simulink model "B5_simulation_paparazzi"  (R2021b)
settings: Solver=VariableStepAuto  StartTime=0.0  StopTime=5.5  FixedStep=0.002  RelTol=1e-3
values from neighbouring files (symbols this model uses):
  coef_sim_1 = tf_des_d.Denominator{1}(2)    [A11_setup_script_pprz.m]    (also in A1_setup_script.m; A6_slow_actuator.m)
  coef_sim_2 = tf_des_d.Numerator{1}(2)    [A11_setup_script_pprz.m]    (also in A1_setup_script.m; A6_slow_actuator.m)
  coeff = 1    [A11_setup_script_pprz.m]    (also in A12_sim_multi_run.m = coeff_list(i))
  doublet_mag = - 0.15    (= -0.15)    [A11_setup_script_pprz.m]    (also in A1_setup_script.m)
  doublet_time = 6    [A11_setup_script_pprz.m]    (also in A1_setup_script.m)
  f_8 = 1    [A11_setup_script_pprz.m]    (also in A1_setup_script.m)
  FILT_CUTOFF = 2*pi*5    (= 31.4159265359)    [A11_setup_script_pprz.m]    (also in A1_setup_script.m)
  FILTER = 1    [A11_setup_script_pprz.m]    (also in A1_setup_script.m)
  G1 = inv(I)*G1_r    [A10_simple_plant.m]    (also in A11_setup_script_pprz.m = G1/scale; A1_setup_script.m = [G1;G1_T])
  G2 = G2/scale    [A11_setup_script_pprz.m]    (also in A1_setup_script.m = (1/sampling_time)*inv(I)*(G2_r))
  h_plate = 0.3    [A11_setup_script_pprz.m]    (also in A1_setup_script.m = 0.16)
  I = eye(3,3)    [A10_simple_plant.m]    (also in A11_setup_script_pprz.m; A1_setup_script.m; A2_B_matrix_generation_symbolic.m = [Ixx 0 0; A3_B_matrix_generation_symbolic_cascaded.m = [Ixx 0 0)
  Iyy = 0.0008    [A11_setup_script_pprz.m]    (also in A1_setup_script.m = 0.0015)
  K = 7    [A11_setup_script_pprz.m]    (also in A1_setup_script.m = 10)
  K_act = 50    [A10_simple_plant.m]    (also in A11_setup_script_pprz.m = 20; A1_setup_script.m = 20)
  K_d = 15    [A11_setup_script_pprz.m]    (also in A1_setup_script.m = 25)
  K_dd = K_act    (= 20)    [A11_setup_script_pprz.m]    (also in A1_setup_script.m)
  K_ec = 50    [A11_setup_script_pprz.m]    (also in A1_setup_script.m = 251)
  K_ec_d = 13    [A11_setup_script_pprz.m]    (also in A1_setup_script.m = 25)
  K_ec_d_u = 1.5    [A11_setup_script_pprz.m]    (also in A1_setup_script.m = 5)
  K_ec_d_v = 1.5    [A11_setup_script_pprz.m]    (also in A1_setup_script.m = 5)
  K_ec_dd = 9    [A11_setup_script_pprz.m]    (also in A1_setup_script.m = 45)
  K_ec_i = 0    [A11_setup_script_pprz.m]    (also in A1_setup_script.m = 380)
  K_ec_u = 1.5    [A11_setup_script_pprz.m]    (also in A1_setup_script.m = 5)
  K_ec_v = 1.5    [A11_setup_script_pprz.m]    (also in A1_setup_script.m = 5)
  K_t = 0.0005    [A10_simple_plant.m]    (also in A11_setup_script_pprz.m = 6.557e-08; A1_setup_script.m = 6.557e-08)
  K_u = 1.0    (= 1)    [A11_setup_script_pprz.m]    (also in A1_setup_script.m = 1.5)
  K_u_d = 2.5    [A11_setup_script_pprz.m]    (also in A1_setup_script.m = 7)
  K_v = 1.0    (= 1)    [A11_setup_script_pprz.m]    (also in A1_setup_script.m = 1.5)
  K_v_d = 2.5    [A11_setup_script_pprz.m]    (also in A1_setup_script.m = 7)
  K_w = 1.0    (= 1)    [A11_setup_script_pprz.m]    (also in A1_setup_script.m = 4.5)
  K_w_d = 2.5    [A11_setup_script_pprz.m]    (also in A1_setup_script.m = 7)
  l_plate = 0.1    [A11_setup_script_pprz.m]    (also in A1_setup_script.m = 0.11)
  m = 0.4    [A10_simple_plant.m]    (also in A11_setup_script_pprz.m; A1_setup_script.m)
  NOISE = 0    [A11_setup_script_pprz.m]    (also in A1_setup_script.m)
  NOISE_ACC = 0.00005    (= 5e-05)    [A11_setup_script_pprz.m]    (also in A1_setup_script.m)
  NOISE_GYRO = 0.00005    (= 5e-05)    [A11_setup_script_pprz.m]    (also in A1_setup_script.m)
  NOISE_RPM = 200    [A11_setup_script_pprz.m]    (also in A1_setup_script.m)
  omega_des = 20.00    (= 20)    [A11_setup_script_pprz.m]    (also in A1_setup_script.m; A6_slow_actuator.m = 49)
  sampling_time = 1/frequency    (= 0.002)    [A11_setup_script_pprz.m]    (also in A12_sim_multi_run.m; A1_setup_script.m; A6_slow_actuator.m)
  scale_8 = 1.6    [A11_setup_script_pprz.m]    (also in A1_setup_script.m)
  start_8 = 2    [A11_setup_script_pprz.m]    (also in A1_setup_script.m)
  start_time = 2    [A11_setup_script_pprz.m]    (also in A1_setup_script.m = 1)
  t_8 = 10    [A11_setup_script_pprz.m]    (also in A1_setup_script.m)
  w_plate = 0.3    [A11_setup_script_pprz.m]    (also in A1_setup_script.m = 0.36)
undefined symbols (not defined in the file or in its folder): DiscIntNeverNeededParam
libraries: simulink x11, cstblocks x9, dspinverses x8, dspmathops x4, dspstat3 x4, aerolibutil x3, sharedutil x2, aerolibanim x1
(part 1 of 5)
settings Model: Creator=pcampolucci  LastModifiedBy=pcampolucci

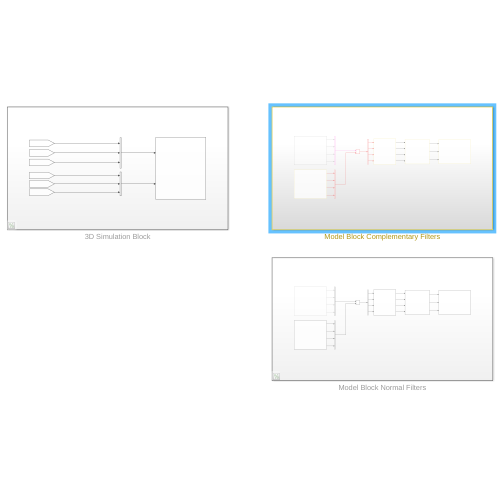
[thumbnail: Simulink's stored preview of the top-level diagram]
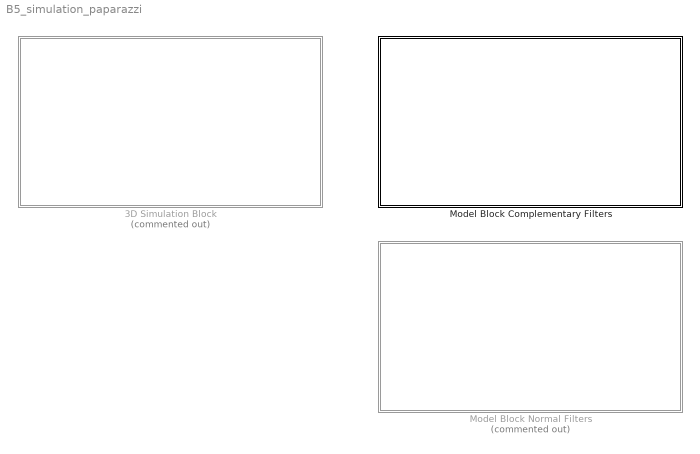
== system B5_simulation_paparazzi ==
  3D Simulation Block : Subsystem  Commented=on
  Model Block Complementary Filters : Subsystem
  Model Block Normal Filters : Subsystem  Commented=on

== system B5_simulation_paparazzi/3D Simulation Block ==
  6DoF Animation : aerolibanim/6DoF Animation  u1=[-4 4 -4 4 -1 1]  u2=0.1  u3=0.3  u4=[0 0 0]  u5=Fly alongside  u6=[5 5 -4]  u7=10  u8=on
  Vector Concatenate : Concatenate  NumInputs=3
  Vector Concatenate1 : Concatenate  NumInputs=3
  wires:
  [psi] -> Vector Concatenate/3
  Vector Concatenate1/1 -> 6DoF Animation/1
  Vector Concatenate/1 -> 6DoF Animation/2
  [X_cont] -> Vector Concatenate1/1
  [Y_cont] -> Vector Concatenate1/2
  [theta] -> Vector Concatenate/2
  [phi] -> Vector Concatenate/1
  [Z_cont] -> Vector Concatenate1/3

== system B5_simulation_paparazzi/Model Block Complementary Filters ==
  Continuous Actuator Dynamics : Subsystem
  Demux : Demux
  Extended INDI : Subsystem
  Force and Moment Calculation : Subsystem
      mask Display: image('/home/pcampolucci/asc-indi-simulator/media/bebop.jpg'); % Use "Edit Image" on toolstrip to change.
  Manual Switch : ManualSwitch
  Mux1 : Mux
  Mux4 : Mux
  Plant and State Estimation : Subsystem
  Simple INDI : Subsystem  Commented=on
  wires:
  Demux/2 -> Continuous Actuator Dynamics/2(Motor_2_omega_input)
  Demux/4 -> Continuous Actuator Dynamics/4(Motor_4_omega_input)
  Continuous Actuator Dynamics/1(omega_1) -> Force and Moment Calculation/1(omega_1)
  Continuous Actuator Dynamics/4(omega_4) -> Force and Moment Calculation/4(omega_4)
  Demux/1 -> Continuous Actuator Dynamics/1(Motor_1_omega_input)
  Force and Moment Calculation/1(Moments in body frame) -> Plant and State Estimation/1(Moments in body frame)
  Continuous Actuator Dynamics/3(omega_3) -> Force and Moment Calculation/3(omega_3)
  Continuous Actuator Dynamics/2(omega_2) -> Force and Moment Calculation/2(omega_2)
  Demux/3 -> Continuous Actuator Dynamics/3(Motor_3_omega_input)
  Force and Moment Calculation/2(Forces in earth frame) -> Plant and State Estimation/2(Forces in earth frame)
  Extended INDI/2(Motor_2_omega_input) -> Mux4/2
  Extended INDI/1(Motor_1_omega_input) -> Mux4/1
  Extended INDI/3(Motor_3_omega_input) -> Mux4/3
  Extended INDI/4(Motor_4_omega_input) -> Mux4/4
  Force and Moment Calculation/3(Collective Thrust) -> Plant and State Estimation/3(Collective Thrust)
  Mux4/1 -> Manual Switch/1
  Manual Switch/1 -> Demux/1
  Simple INDI/1(Motor_1_omega_input) -> Mux1/1
  Simple INDI/2(Motor_2_omega_input) -> Mux1/2
  Simple INDI/3(Motor_3_omega_input) -> Mux1/3
  Simple INDI/4(Motor_4_omega_input) -> Mux1/4
  Mux1/1 -> Manual Switch/2

== system B5_simulation_paparazzi/Model Block Normal Filters ==
  Continuous Actuator Dynamics : Subsystem
  Demux : Demux
  Extended INDI : Subsystem  Commented=on
  Force and Moment Calculation : Subsystem
      mask Display: image('/home/pcampolucci/asc-indi-simulator/media/bebop.jpg'); % Use "Edit Image" on toolstrip to change.
  Manual Switch : ManualSwitch  CurrentSetting=0
  Mux1 : Mux
  Mux4 : Mux
  Plant and State Estimation : Subsystem
  Simple INDI : Subsystem
  wires:
  Demux/2 -> Continuous Actuator Dynamics/2(Motor_2_omega_input)
  Demux/4 -> Continuous Actuator Dynamics/4(Motor_4_omega_input)
  Continuous Actuator Dynamics/1(omega_1) -> Force and Moment Calculation/1(omega_1)
  Continuous Actuator Dynamics/4(omega_4) -> Force and Moment Calculation/4(omega_4)
  Demux/1 -> Continuous Actuator Dynamics/1(Motor_1_omega_input)
  Force and Moment Calculation/1(Moments in body frame) -> Plant and State Estimation/1(Moments in body frame)
  Continuous Actuator Dynamics/3(omega_3) -> Force and Moment Calculation/3(omega_3)
  Continuous Actuator Dynamics/2(omega_2) -> Force and Moment Calculation/2(omega_2)
  Demux/3 -> Continuous Actuator Dynamics/3(Motor_3_omega_input)
  Force and Moment Calculation/2(Forces in earth frame) -> Plant and State Estimation/2(Forces in earth frame)
  Extended INDI/2(Motor_2_omega_input) -> Mux4/2
  Extended INDI/1(Motor_1_omega_input) -> Mux4/1
  Extended INDI/3(Motor_3_omega_input) -> Mux4/3
  Extended INDI/4(Motor_4_omega_input) -> Mux4/4
  Force and Moment Calculation/3(Collective Thrust) -> Plant and State Estimation/3(Collective Thrust)
  Mux4/1 -> Manual Switch/1
  Manual Switch/1 -> Demux/1
  Simple INDI/1(Motor_1_omega_input) -> Mux1/1
  Simple INDI/2(Motor_2_omega_input) -> Mux1/2
  Simple INDI/3(Motor_3_omega_input) -> Mux1/3
  Simple INDI/4(Motor_4_omega_input) -> Mux1/4
  Mux1/1 -> Manual Switch/2

== system B5_simulation_paparazzi/Model Block Complementary Filters/Continuous Actuator Dynamics ==
  Motor_1_omega_input : Inport
  Motor_2_omega_input : Inport  Port=2
  Motor_3_omega_input : Inport  Port=3
  Motor_4_omega_input : Inport  Port=4
  Demux : Demux
  Discrete Transfer Fcn{1..4} (4 alike) : DiscreteTransferFcn  Numerator=[coef_sim_2]  Denominator=[1 coef_sim_1]  SampleTime=sampling_time
  Mux : Mux
  Noise RPM : Subsystem
  Sum : Sum  Inputs=|++
  Transfer Fcn{,1..3} (4 alike) : TransferFcn  Numerator=[omega_des]  Denominator=[1 omega_des]
  omega_1 : Outport
  omega_2 : Outport  Port=2
  omega_3 : Outport  Port=3
  omega_4 : Outport  Port=4
  tag scope: omega_1_f=global, omega_2_f=global, omega_3_f=global, omega_4_f=global
  wires:
  Transfer Fcn3/1 -> omega_4/1  "omega_4"
  Motor_4_omega_input/1 -> Transfer Fcn3/1, Discrete Transfer Fcn4/1  "omega_4_in"
  Motor_3_omega_input/1 -> Transfer Fcn2/1, Discrete Transfer Fcn3/1  "omega_3_in"
  Transfer Fcn1/1 -> omega_2/1  "omega_2"
  Discrete Transfer Fcn2/1 -> Mux/1
  Motor_2_omega_input/1 -> Transfer Fcn1/1, Discrete Transfer Fcn1/1  "omega_2_in"
  Demux/2 -> [omega_2_f]  "omega_2_est"
  Motor_1_omega_input/1 -> Discrete Transfer Fcn2/1, Transfer Fcn/1  "omega_1_in"
  Transfer Fcn/1 -> omega_1/1  "omega_1"
  Demux/4 -> [omega_4_f]  "omega_4_est"
  Discrete Transfer Fcn4/1 -> Mux/4
  Discrete Transfer Fcn1/1 -> Mux/2
  Discrete Transfer Fcn3/1 -> Mux/3
  Transfer Fcn2/1 -> omega_3/1  "omega_3"
  Demux/1 -> [omega_1_f]  "omega_1_est"
  Demux/3 -> [omega_3_f]  "omega_3_est"
  Mux/1 -> Sum/1  "pqr_measured"
  Noise RPM/1(Out) -> Sum/2
  Sum/1 -> Demux/1

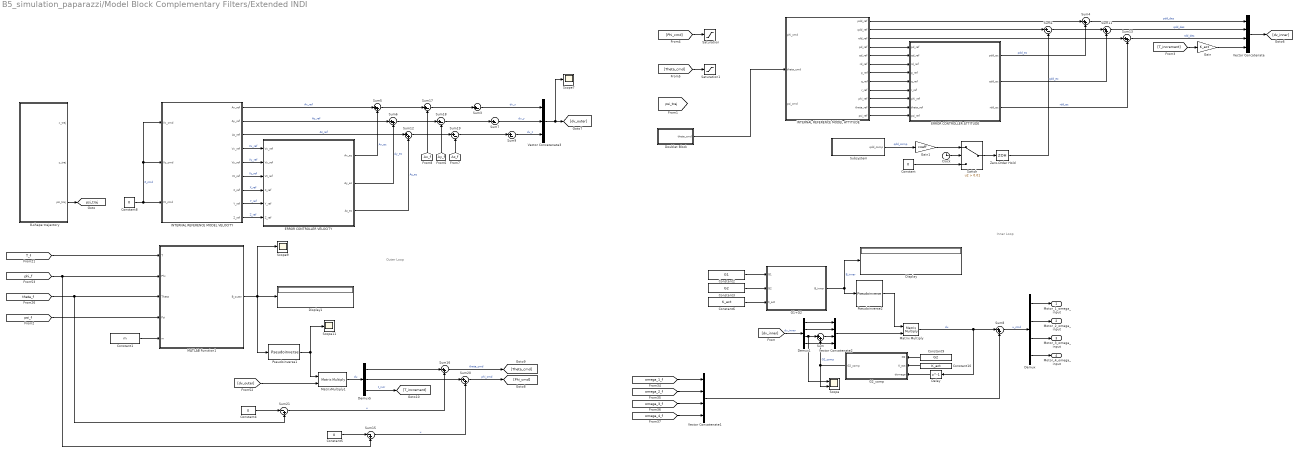
== system B5_simulation_paparazzi/Model Block Complementary Filters/Extended INDI ==
  note: Inner Loop
  note: Outer Loop
  8-shape trajectory : Subsystem
  Clock : Clock
  Constant : Constant  Value=0  SampleTime=sampling_time
  Constant1 : Constant  Value=m  SampleTime=sampling_time
  Constant10 : Constant  Value=K_act  SampleTime=sampling_time
  Constant2 : Constant  Value=G1  SampleTime=sampling_time
  Constant3 : Constant  Value=G2  SampleTime=sampling_time
  Constant4 : Constant  Value=0
  Constant5 : Constant  Value=0
  Constant6 : Constant  Value=K_act  SampleTime=sampling_time
  Constant8 : Constant  Value=0  SampleTime=sampling_time
  Constant9 : Constant  Value=G2  SampleTime=sampling_time
  Delay : Delay  DelayLength=1
  Demux : Demux
  Demux1 : Demux
  Demux5 : Demux  Outputs=3
  Display : Display
  Display1 : Display
  Doublet Block : Subsystem
  ERROR CONTROLLER ATTITUDE : Subsystem
  ERROR CONTROLLER VELOCITY : Subsystem
  G1+G2 : MATLAB Function  TreatAsAtomicUnit=on
  G2_comp : MATLAB Function  TreatAsAtomicUnit=on
  Gain : Gain  Gain=K_act
  Gain1 : Gain  Gain=coeff
  INTERNAL REFERENCE MODEL ATTITUDE : Subsystem
  INTERNAL REFERENCE MODEL VELOCITY : Subsystem
  MATLAB Function1 : MATLAB Function  TreatAsAtomicUnit=on
  Matrix Multiply : Product  Multiplication=Matrix(*)
  MatrixMultiply1 : Product  Multiplication=Matrix(*)
  Pseudoinverse1 : dspinverses/Pseudoinverse  wanterr=off  SimulateUsing=Interpreted execution
      settings: SourceProductBaseCode=DS
  Pseudoinverse2 : dspinverses/Pseudoinverse  wanterr=off  SimulateUsing=Interpreted execution
      settings: SourceProductBaseCode=DS
  Saturation : Saturate
  Saturation1 : Saturate
  Scope : Scope  NumInputPorts=2
  Scope11 : Scope
  Scope7 : Scope
  Scope9 : Scope
  Subsystem : Subsystem
  Sum{,4..6,8,11..13,16,20} (10 alike) : Sum  Inputs=|++
  Sum{1,3,7,9,17..19} (7 alike) : Sum  Inputs=|+-
  Sum15 : Sum  Inputs=|-+
  Sum21 : Sum  Inputs=|-+
  Switch : Switch  Criteria=u2 > Threshold  Threshold=0.01
  Vector Concatenate : Concatenate  NumInputs=4
  Vector Concatenate1 : Concatenate  NumInputs=4
  Vector Concatenate2 : Concatenate  NumInputs=4
  Vector Concatenate3 : Concatenate  NumInputs=3
  Zero-Order Hold : ZeroOrderHold  SampleTime=sampling_time
  Motor_1_omega_input : Outport
  Motor_2_omega_input : Outport  Port=2
  Motor_3_omega_input : Outport  Port=3
  Motor_4_omega_input : Outport  Port=4
  tag scope: psi_traj=global
  wires:
  G1+G2/1(B_inner) -> Pseudoinverse2/1, Display/1  "B_inner"
  Vector Concatenate/1 -> [dv_inner]
  Matrix Multiply/1 -> Delay/1, Sum8/1  "du"
  Demux/1 -> Motor_1_omega_input/1
  [omega_4_f] -> Vector Concatenate1/4
  [omega_2_f] -> Vector Concatenate1/2
  Demux/3 -> Motor_3_omega_input/1
  Sum8/1 -> Demux/1  "u_cmd"
  Pseudoinverse2/1 -> Matrix Multiply/1
  [omega_1_f] -> Vector Concatenate1/1
  Demux/2 -> Motor_2_omega_input/1
  Demux/4 -> Motor_4_omega_input/1
  [omega_3_f] -> Vector Concatenate1/3
  INTERNAL REFERENCE MODEL VELOCITY/5(Vy_ref) -> ERROR CONTROLLER VELOCITY/2(Vy_ref)  "Vy_ref"
  Constant4/1 -> Sum21/1
  Sum16/1 -> [Theta_cmd]  "theta_cmd"
  Sum9/1 -> Vector Concatenate3/3  "dv_z"
  INTERNAL REFERENCE MODEL VELOCITY/2(Ay_ref) -> Sum6/1  "Ay_ref"
  Sum21/1 -> Sum16/2  "u"
  INTERNAL REFERENCE MODEL VELOCITY/6(Vz_ref) -> ERROR CONTROLLER VELOCITY/3(Vz_ref)  "Vz_ref"
  INTERNAL REFERENCE MODEL VELOCITY/4(Vx_ref) -> ERROR CONTROLLER VELOCITY/1(Vx_ref)  "Vx_ref"
  ERROR CONTROLLER VELOCITY/2(Ay_ec) -> Sum6/2  "Ay_ec"
  Sum7/1 -> Vector Concatenate3/2  "dv_y"
  ERROR CONTROLLER VELOCITY/1(Ax_ec) -> Sum5/2  "Ax_ec"
  Sum3/1 -> Vector Concatenate3/1  "dv_x"
  ERROR CONTROLLER VELOCITY/3(Az_ec) -> Sum12/2  "Az_ec"
  Sum12/1 -> Sum19/1
  Constant8/1 -> INTERNAL REFERENCE MODEL VELOCITY/2(Vy_cmd), INTERNAL REFERENCE MODEL VELOCITY/1(Vx_cmd), INTERNAL REFERENCE MODEL VELOCITY/3(Vz_cmd)  "Z_cmd"
  Pseudoinverse1/1 -> Scope11/1, MatrixMultiply1/1
  Sum15/1 -> Sum20/2  "u"
  Vector Concatenate3/1 -> Scope7/1, [dv_outer]
  INTERNAL REFERENCE MODEL VELOCITY/1(Ax_ref) -> Sum5/1  "Ax_ref"
  INTERNAL REFERENCE MODEL VELOCITY/3(Az_ref) -> Sum12/1  "Az_ref"
  Sum20/1 -> [Phi_cmd]  "phi_cmd"
  [T_f] -> MATLAB Function1/1(T)
  Sum6/1 -> Sum18/1
  Constant5/1 -> Sum15/1
  [dv_outer] -> MatrixMultiply1/2
  MATLAB Function1/1(B_outer) -> Scope9/1, Display1/1, Pseudoinverse1/1
  Demux5/3 -> [T_increment]  "t_incr"
  MatrixMultiply1/1 -> Demux5/1  "du"
  [T_increment] -> Gain/1
  [Ax_f] -> Sum17/2
  [Ay_f] -> Sum18/2
  [Az_f] -> Sum19/2
  [Phi_cmd] -> Saturation/1
  [theta_f] -> Sum21/2, MATLAB Function1/3(Theta)
  [phi_f] -> Sum15/2, MATLAB Function1/2(Phi)
  INTERNAL REFERENCE MODEL ATTITUDE/4(pd_ref) -> ERROR CONTROLLER ATTITUDE/1(pd_ref)
  INTERNAL REFERENCE MODEL ATTITUDE/7(p_ref) -> ERROR CONTROLLER ATTITUDE/4(p_ref)
  ERROR CONTROLLER ATTITUDE/3(rdd_ec) -> Sum13/2  "rdd_ec"
  ERROR CONTROLLER ATTITUDE/2(qdd_ec) -> Sum11/2  "qdd_ec"
  INTERNAL REFERENCE MODEL ATTITUDE/5(qd_ref) -> ERROR CONTROLLER ATTITUDE/2(qd_ref)
  INTERNAL REFERENCE MODEL ATTITUDE/11(theta_ref) -> ERROR CONTROLLER ATTITUDE/8(theta_ref)
  INTERNAL REFERENCE MODEL ATTITUDE/1(pdd_ref) -> Sum4/1
  INTERNAL REFERENCE MODEL ATTITUDE/8(q_ref) -> ERROR CONTROLLER ATTITUDE/5(q_ref)
  ERROR CONTROLLER ATTITUDE/1(pdd_ec) -> Sum4/2  "pdd_ec"
  INTERNAL REFERENCE MODEL ATTITUDE/6(rd_ref) -> ERROR CONTROLLER ATTITUDE/3(rd_ref)
  INTERNAL REFERENCE MODEL ATTITUDE/10(phi_ref) -> ERROR CONTROLLER ATTITUDE/7(phi_ref)
  INTERNAL REFERENCE MODEL ATTITUDE/12(psi_ref) -> ERROR CONTROLLER ATTITUDE/9(psi_ref)
  INTERNAL REFERENCE MODEL ATTITUDE/9(r_ref) -> ERROR CONTROLLER ATTITUDE/6(r_ref)
  Sum13/1 -> Vector Concatenate/3  "rdd_des"
  Sum4/1 -> Vector Concatenate/1  "pdd_des"
  Sum11/1 -> Vector Concatenate/2  "qdd_des"
  Gain/1 -> Vector Concatenate/4
  Constant3/1 -> G1+G2/2(G2)
  Constant6/1 -> G1+G2/3(K_act)
  Constant2/1 -> G1+G2/1(G1)
  Constant9/1 -> G2_comp/1(G2)
  Constant10/1 -> G2_comp/2(K_act)
  [dv_inner] -> Demux1/1  "dv_inner"
  Sum/1 -> Vector Concatenate2/3
  Demux1/3 -> Scope/1, Sum/1
  Demux1/2 -> Vector Concatenate2/2
  Demux1/1 -> Vector Concatenate2/1
  Demux1/4 -> Vector Concatenate2/4
  Vector Concatenate2/1 -> Matrix Multiply/2
  G2_comp/1(G2_comp) -> Sum/2, Scope/2  "G2_comp"
  Sum5/1 -> Sum17/1
  INTERNAL REFERENCE MODEL ATTITUDE/2(qdd_ref) -> Sum1/1
  8-shape trajectory/3(psi_traj) -> [psi_traj]
  [Theta_cmd] -> Saturation1/1
  Sum17/1 -> Sum3/1
  Sum18/1 -> Sum7/1
  Sum19/1 -> Sum9/1
  Constant1/1 -> MATLAB Function1/5(m)
  Demux5/2 -> Sum20/1
  Demux5/1 -> Sum16/1
  [psi_f] -> MATLAB Function1/4(Psi)
  Clock/1 -> Switch/2
  Constant/1 -> Switch/3
  Switch/1 -> Zero-Order Hold/1
  INTERNAL REFERENCE MODEL VELOCITY/7(X_ref) -> ERROR CONTROLLER VELOCITY/4(X_ref)  "X_ref"
  INTERNAL REFERENCE MODEL VELOCITY/8(Y_ref) -> ERROR CONTROLLER VELOCITY/5(Y_ref)  "Y_ref"
  INTERNAL REFERENCE MODEL VELOCITY/9(Z_ref) -> ERROR CONTROLLER VELOCITY/6(Z_ref)  "Z_ref"
  Doublet Block/1(theta_cmd) -> INTERNAL REFERENCE MODEL ATTITUDE/2(theta_cmd)
  INTERNAL REFERENCE MODEL ATTITUDE/3(rdd_ref) -> Sum13/1
  Subsystem/1(qdd_comp) -> Gain1/1  "qdd_comp"
  Sum1/1 -> Sum11/1
  Zero-Order Hold/1 -> Sum1/2
  Gain1/1 -> Switch/1
  Vector Concatenate1/1 -> Sum8/2
  Delay/1 -> G2_comp/3(domega)

== system B5_simulation_paparazzi/Model Block Complementary Filters/Force and Moment Calculation ==
  omega_1 : Inport
  omega_2 : Inport  Port=2
  omega_3 : Inport  Port=3
  omega_4 : Inport  Port=4
  Add : Sum
  Add1 : Sum
  Constant : Constant  Value=0
  Constant1 : Constant  Value=sampling_time  SampleTime=sampling_time
  Constant2 : Constant  Value=G1  SampleTime=sampling_time
  Constant3 : Constant  Value=G2  SampleTime=sampling_time
  Constant5 : Constant  Value=I  SampleTime=sampling_time
  Derivative : Derivative
  Drag Plate Aerodynamics : Subsystem
  Forces due to thrust : MATLAB Function  TreatAsAtomicUnit=on
  Gain : Gain  Gain=0.09
  Gain1 : Gain  Gain=0.09
  Moments due to thrust : MATLAB Function  TreatAsAtomicUnit=on
  Mux : Mux
  Mux1 : Mux  Inputs=3
  Sum : Sum  Inputs=|++
  Moments in body frame : Outport
  Forces in earth frame : Outport  Port=2
  Collective Thrust : Outport  Port=3
  wires:
  Moments due to thrust/1(M_t) -> Add1/2  "thrust_moment_in"
  Constant2/1 -> Forces due to thrust/3(G1), Moments due to thrust/3(G1)
  Constant3/1 -> Moments due to thrust/4(G2)
  omega_4/1 -> Mux/4
  omega_3/1 -> Mux/3
  omega_2/1 -> Mux/2
  omega_1/1 -> Mux/1
  Mux/1 -> Derivative/1, Forces due to thrust/1(omega), Moments due to thrust/1(omega)
  Derivative/1 -> Moments due to thrust/2(omega_dot)
  Constant1/1 -> Moments due to thrust/5(sampling_time)
  [R_bg] -> Forces due to thrust/2(R_bg)
  Forces due to thrust/1(F_t_e) -> Add/2  "thrust_earth"
  Forces due to thrust/2(F_t_b) -> Collective Thrust/1  "thrust_body"
  Add/1 -> Forces in earth frame/1
  Add1/1 -> Moments in body frame/1  "full_moment_in"
  Constant5/1 -> Moments due to thrust/6(I)
  Drag Plate Aerodynamics/1(aero_moment) -> Add1/1  "aero_moment_in"
  Constant/1 -> Mux1/3, Mux1/1
  [theta_cont] -> Gain/1
  [phi_cont] -> Gain1/1
  Gain/1 -> Sum/1
  Gain1/1 -> Sum/2
  Sum/1 -> Mux1/2
  Mux1/1 -> ?  "dummy_moment"

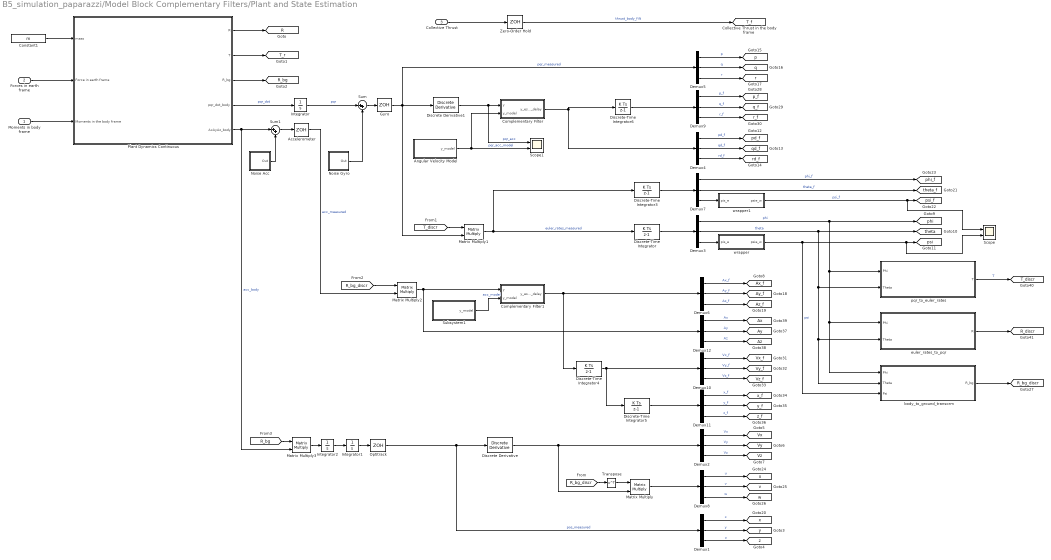
== system B5_simulation_paparazzi/Model Block Complementary Filters/Plant and State Estimation ==
  Moments in body frame : Inport
  Forces in earth frame : Inport  Port=2
  Collective Thrust : Inport  Port=3
  Accelerometer : ZeroOrderHold  SampleTime=sampling_time
  Angular Velocity Model : Subsystem
  Complementary Filter : Subsystem
  Complementary Filter1 : Subsystem
  Constant1 : Constant  Value=m  SampleTime=sampling_time
  Demux{1..12} (12 alike) : Demux  Outputs=3
  Discrete Derivative : simulink/Discrete/Discrete Derivative  gainval=1.0  ICPrevScaledInput=0.0  OutMin=[]  OutMax=[]  OutDataType=fixdt(1, 16)  OutScaling=2^-10  DoSatur=off
  Discrete Derivative1 : simulink/Discrete/Discrete Derivative  gainval=1.0  ICPrevScaledInput=0.0  OutMin=[]  OutMax=[]  OutDataType=fixdt(1, 16)  OutScaling=2^-10  DoSatur=off
  Discrete-Time Integrator{,3..5} (4 alike) : DiscreteIntegrator  SampleTime=sampling_time  ICPrevOutput=DiscIntNeverNeededParam  ICPrevScaledInput=DiscIntNeverNeededParam
  Discrete-Time Integrator6 : DiscreteIntegrator  SampleTime=-1  ICPrevOutput=DiscIntNeverNeededParam  ICPrevScaledInput=DiscIntNeverNeededParam
  Gyro : ZeroOrderHold  SampleTime=sampling_time
  Integrator : Integrator
  Integrator1 : Integrator
  Integrator2 : Integrator
  Matrix Multiply{,1..3} (4 alike) : Product  Multiplication=Matrix(*)
  Noise Acc : Subsystem
  Noise Gyro : Subsystem
  Optitrack : ZeroOrderHold  SampleTime=sampling_time
  Plant Dynamics Continuous : Subsystem
  Scope : Scope  NumInputPorts=2
  Scope1 : Scope  NumInputPorts=2
  Subsystem1 : Subsystem
  Sum : Sum  Inputs=|++
  Sum1 : Sum  Inputs=|++
  Transpose : Math  Operator=transpose  SaturateOnIntegerOverflow=on
  Zero-Order Hold : ZeroOrderHold  SampleTime=sampling_time
  body_to_ground_transorm : MATLAB Function  Description=|  TreatAsAtomicUnit=on
      | This function computes the rotational matrix to pass from the body frame to the world frame. 
      | Takes as inpout the euler angles.
  euler_rates_to_pqr : MATLAB Function  TreatAsAtomicUnit=on
  pqr_to_euler_rates : MATLAB Function  TreatAsAtomicUnit=on
  wrapper : MATLAB Function  TreatAsAtomicUnit=on
  wrapper1 : MATLAB Function  TreatAsAtomicUnit=on
  tag scope: Ax=global, Ax_f=global, Ay=global, Ay_f=global, Az=global, Az_f=global, R=global, R_bg=global, R_bg_discr=global, R_discr=global, T_discr=global, T_f=global, T_r=global, Vx=global, Vx_f=global, Vy=global, Vy_f=global, Vz=global, Vz_f=global, p=global, p_f=global, pd_f=global, phi=global, phi_f=global, psi=global, psi_f=global, q=global, q_f=global, qd_f=global, r=global, r_f=global, rd_f=global, theta=global, theta_f=global, u=global, v=global, w=global, x=global, x_f=global, y=global, y_f=global, z=global, z_f=global
  wires:
  Demux3/2 -> euler_rates_to_pqr/2(Theta), body_to_ground_transorm/2(Theta), pqr_to_euler_rates/2(Theta), [theta]  "theta"
  Demux4/1 -> [pd_f]  "pd_f"
  Demux3/1 -> body_to_ground_transorm/1(Phi), euler_rates_to_pqr/1(Phi), pqr_to_euler_rates/1(Phi), [phi]  "phi"
  Demux4/2 -> [qd_f]  "qd_f"
  Demux3/3 -> wrapper/1(pis_e)
  Discrete-Time Integrator/1 -> Demux3/1
  Demux5/2 -> [q]  "q"
  Demux5/1 -> [p]  "p"
  Plant Dynamics Continuous/4(pqr_dot_body) -> Integrator/1  "pqr_dot"
  Demux5/3 -> [r]  "r"
  Integrator/1 -> Sum/1  "pqr"
  Complementary Filter/1(y_est_no_delay) -> Discrete-Time Integrator6/1, Demux4/1
  Demux4/3 -> [rd_f]  "rd_f"
  Moments in body frame/1 -> Plant Dynamics Continuous/3(Moments in the body frame)
  Constant1/1 -> Plant Dynamics Continuous/1(mass)
  Forces in earth frame/1 -> Plant Dynamics Continuous/2(Force in earth frame)
  Plant Dynamics Continuous/1(R) -> [R]
  Plant Dynamics Continuous/2(T) -> [T_r]
  Plant Dynamics Continuous/3(R_bg) -> [R_bg]
  Demux2/2 -> [Vy]  "Vy"
  Demux6/2 -> [Ay_f]  "Ay_f"
  Discrete Derivative/1 -> Demux2/1, Matrix Multiply/2
  Demux6/1 -> [Ax_f]  "Ax_f"
  Accelerometer/1 -> Matrix Multiply2/2  "acc_measured"
  Demux2/1 -> [Vx]  "Vx"
  Demux1/2 -> [y]  "y"
  Demux1/1 -> [x]  "x"
  Demux1/3 -> [z]  "z"
  Demux6/3 -> [Az_f]  "Az_f"
  Demux2/3 -> [Vz]  "Vz"
  Plant Dynamics Continuous/5(AxAyAz_body) -> Matrix Multiply3/2, Sum1/1  "acc_body"
  Demux7/3 -> wrapper1/1(pis_e)
  Demux7/1 -> [phi_f]  "phi_f"
  Demux7/2 -> [theta_f]  "theta_f"
  Discrete-Time Integrator3/1 -> Demux7/1
  [R_bg_discr] -> Transpose/1
  Transpose/1 -> Matrix Multiply/1
  Demux8/2 -> [v]  "v"
  Demux8/1 -> [u]  "u"
  Demux8/3 -> [w]  "w"
  Matrix Multiply/1 -> Demux8/1
  Zero-Order Hold/1 -> [T_f]  "thrust_body_filt"
  Collective Thrust/1 -> Zero-Order Hold/1
  Demux9/3 -> [r_f]  "r_f"
  Demux9/1 -> [p_f]  "p_f"
  Demux9/2 -> [q_f]  "q_f"
  Demux10/1 -> [Vx_f]  "Vx_f"
  Demux10/2 -> [Vy_f]  "Vy_f"
  Demux10/3 -> [Vz_f]  "Vz_f"
  Demux11/2 -> [y_f]  "y_f"
  Discrete-Time Integrator5/1 -> Demux11/1
  Demux11/1 -> [x_f]  "x_f"
  Demux11/3 -> [z_f]  "z_f"
  Discrete-Time Integrator4/1 -> Demux10/1, Discrete-Time Integrator5/1
  Demux12/2 -> [Ay]  "Ay"
  Demux12/1 -> [Ax]  "Ax"
  Demux12/3 -> [Az]  "Az"
  [T_discr] -> Matrix Multiply1/1
  Matrix Multiply1/1 -> Discrete-Time Integrator3/1, Discrete-Time Integrator/1  "euler_rates_measured"
  euler_rates_to_pqr/1(R) -> [R_discr]
  pqr_to_euler_rates/1(T) -> [T_discr]  "T"
  body_to_ground_transorm/1(R_bg) -> [R_bg_discr]
  wrapper/1(psie_w) -> body_to_ground_transorm/3(Psi), Scope/2, [psi]  "psi"
  wrapper1/1(psie_w) -> Scope/1, [psi_f]  "psi_f"
  Sum/1 -> Gyro/1
  Sum1/1 -> Accelerometer/1
  Complementary Filter1/1(y_est_no_delay) -> Discrete-Time Integrator4/1, Demux6/1
  Subsystem1/1(y_model) -> Complementary Filter1/2(y_model)  "acc_model"
  Angular Velocity Model/1(y_model) -> Complementary Filter/2(y_model), Scope1/2  "pqr_acc_model"
  [R_bg_discr] -> Matrix Multiply2/1
  Matrix Multiply2/1 -> Complementary Filter1/1(y), Demux12/1
  Discrete Derivative1/1 -> Scope1/1, Complementary Filter/1(y)  "pqr_acc"
  Discrete-Time Integrator6/1 -> Demux9/1
  Gyro/1 -> Demux5/1, Discrete Derivative1/1, Matrix Multiply1/2  "pqr_measured"
  Integrator1/1 -> Optitrack/1
  Integrator2/1 -> Integrator1/1
  Optitrack/1 -> Demux1/1, Discrete Derivative/1  "pos_measured"
  Matrix Multiply3/1 -> Integrator2/1
  [R_bg] -> Matrix Multiply3/1
  Noise Acc/1(Out) -> Sum1/2
  Noise Gyro/1(Out) -> Sum/2

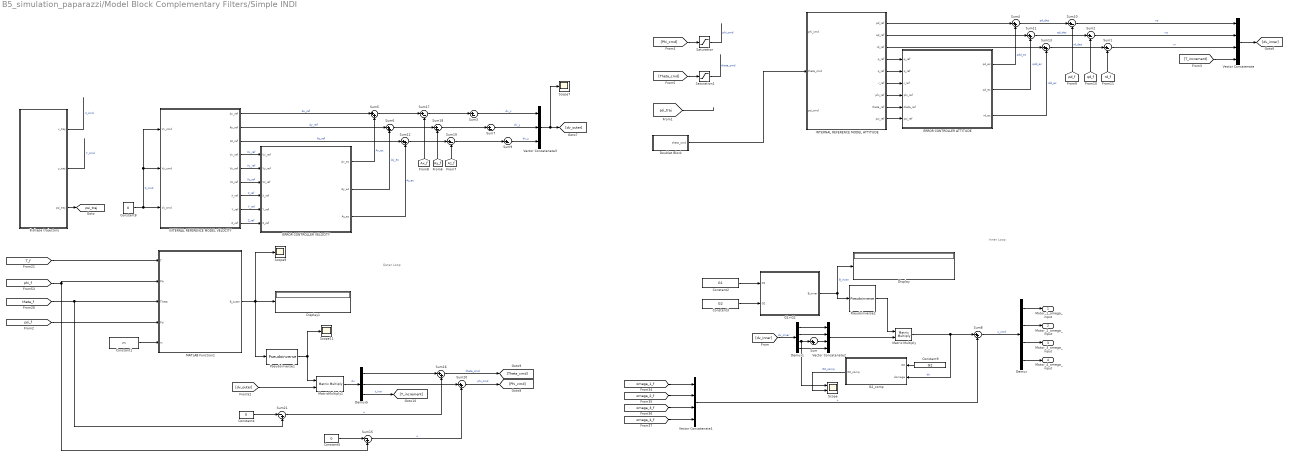
== system B5_simulation_paparazzi/Model Block Complementary Filters/Simple INDI ==
  note: Inner Loop
  note: Outer Loop
  8-shape trajectory : Subsystem
  Constant1 : Constant  Value=m  SampleTime=sampling_time
  Constant2 : Constant  Value=G1  SampleTime=sampling_time
  Constant3 : Constant  Value=G2  SampleTime=sampling_time
  Constant4 : Constant  Value=0
  Constant5 : Constant  Value=0
  Constant8 : Constant  Value=0  SampleTime=sampling_time
  Constant9 : Constant  Value=G2  SampleTime=sampling_time
  Demux : Demux
  Demux1 : Demux
  Demux5 : Demux  Outputs=3
  Display : Display
  Display1 : Display
  Doublet Block : Subsystem
  ERROR CONTROLLER ATTITUDE : Subsystem
  ERROR CONTROLLER VELOCITY : Subsystem
  G1+G2 : MATLAB Function  TreatAsAtomicUnit=on
  G2_comp : MATLAB Function  TreatAsAtomicUnit=on
  INTERNAL REFERENCE MODEL ATTITUDE : Subsystem
  INTERNAL REFERENCE MODEL VELOCITY : Subsystem
  MATLAB Function1 : MATLAB Function  TreatAsAtomicUnit=on
  Matrix Multiply : Product  Multiplication=Matrix(*)
  MatrixMultiply1 : Product  Multiplication=Matrix(*)
  Pseudoinverse1 : dspinverses/Pseudoinverse  wanterr=off  SimulateUsing=Interpreted execution
      settings: SourceProductBaseCode=DS
  Pseudoinverse2 : dspinverses/Pseudoinverse  wanterr=off  SimulateUsing=Interpreted execution
      settings: SourceProductBaseCode=DS
  Saturation : Saturate
  Saturation1 : Saturate
  Scope : Scope  NumInputPorts=2
  Scope11 : Scope
  Scope7 : Scope
  Scope9 : Scope
  Sum{,4..6,8,11..13,16,20} (10 alike) : Sum  Inputs=|++
  Sum{1..3,7,9..10,17..19} (9 alike) : Sum  Inputs=|+-
  Sum15 : Sum  Inputs=|-+
  Sum21 : Sum  Inputs=|-+
  Vector Concatenate : Concatenate  NumInputs=4
  Vector Concatenate1 : Concatenate  NumInputs=4
  Vector Concatenate2 : Concatenate  NumInputs=4
  Vector Concatenate3 : Concatenate  NumInputs=3
  Motor_1_omega_input : Outport
  Motor_2_omega_input : Outport  Port=2
  Motor_3_omega_input : Outport  Port=3
  Motor_4_omega_input : Outport  Port=4
  tag scope: psi_traj=global
  wires:
  G1+G2/1(B_inner) -> Pseudoinverse2/1, Display/1  "B_inner"
  Vector Concatenate1/1 -> Sum8/2  "u"
  Vector Concatenate/1 -> [dv_inner]
  Matrix Multiply/1 -> G2_comp/2(domega), Sum8/1  "du"
  Demux/1 -> Motor_1_omega_input/1
  [omega_4_f] -> Vector Concatenate1/4
  [omega_2_f] -> Vector Concatenate1/2
  Demux/3 -> Motor_3_omega_input/1
  Sum8/1 -> Demux/1  "u_cmd"
  Pseudoinverse2/1 -> Matrix Multiply/1
  [omega_1_f] -> Vector Concatenate1/1
  Demux/2 -> Motor_2_omega_input/1
  Demux/4 -> Motor_4_omega_input/1
  [omega_3_f] -> Vector Concatenate1/3
  INTERNAL REFERENCE MODEL VELOCITY/5(Vy_ref) -> ERROR CONTROLLER VELOCITY/2(Vy_ref)  "Vy_ref"
  Constant4/1 -> Sum21/1
  Sum16/1 -> [Theta_cmd]  "theta_cmd"
  Sum9/1 -> Vector Concatenate3/3  "dv_z"
  INTERNAL REFERENCE MODEL VELOCITY/2(Ay_ref) -> Sum6/1  "Ay_ref"
  Sum21/1 -> Sum16/2  "u"
  INTERNAL REFERENCE MODEL VELOCITY/6(Vz_ref) -> ERROR CONTROLLER VELOCITY/3(Vz_ref)  "Vz_ref"
  INTERNAL REFERENCE MODEL VELOCITY/4(Vx_ref) -> ERROR CONTROLLER VELOCITY/1(Vx_ref)  "Vx_ref"
  ERROR CONTROLLER VELOCITY/2(Ay_ec) -> Sum6/2  "Ay_ec"
  8-shape trajectory/1(x_traj) -> ?  "X_cmd"
  Sum7/1 -> Vector Concatenate3/2  "dv_y"
  ERROR CONTROLLER VELOCITY/1(Ax_ec) -> Sum5/2  "Ax_ec"
  Sum3/1 -> Vector Concatenate3/1  "dv_x"
  ERROR CONTROLLER VELOCITY/3(Az_ec) -> Sum12/2  "Az_ec"
  Sum12/1 -> Sum19/1
  Constant8/1 -> INTERNAL REFERENCE MODEL VELOCITY/1(Vx_cmd), INTERNAL REFERENCE MODEL VELOCITY/2(Vy_cmd), INTERNAL REFERENCE MODEL VELOCITY/3(Vz_cmd)  "Z_cmd"
  Pseudoinverse1/1 -> Scope11/1, MatrixMultiply1/1
  Sum15/1 -> Sum20/2  "u"
  Vector Concatenate3/1 -> Scope7/1, [dv_outer]
  INTERNAL REFERENCE MODEL VELOCITY/1(Ax_ref) -> Sum5/1  "Ax_ref"
  INTERNAL REFERENCE MODEL VELOCITY/3(Az_ref) -> Sum12/1  "Az_ref"
  Sum20/1 -> [Phi_cmd]  "phi_cmd"
  [T_f] -> MATLAB Function1/1(T)
  Sum6/1 -> Sum18/1
  Constant5/1 -> Sum15/1
  [dv_outer] -> MatrixMultiply1/2
  MATLAB Function1/1(B_outer) -> Scope9/1, Display1/1, Pseudoinverse1/1
  Demux5/3 -> [T_increment]  "t_incr"
  MatrixMultiply1/1 -> Demux5/1  "du"
  8-shape trajectory/2(y_traj) -> ?  "Y_cmd"
  [Ax_f] -> Sum17/2
  [Ay_f] -> Sum18/2
  [Az_f] -> Sum19/2
  [Phi_cmd] -> Saturation/1
  [theta_f] -> Sum21/2, MATLAB Function1/3(Theta)
  [phi_f] -> Sum15/2, MATLAB Function1/2(Phi)
  INTERNAL REFERENCE MODEL ATTITUDE/4(p_ref) -> ERROR CONTROLLER ATTITUDE/1(p_ref)
  ERROR CONTROLLER ATTITUDE/3(rd_ec) -> Sum13/2  "rdd_ec"
  ERROR CONTROLLER ATTITUDE/2(qd_ec) -> Sum11/2  "qdd_ec"
  INTERNAL REFERENCE MODEL ATTITUDE/8(theta_ref) -> ERROR CONTROLLER ATTITUDE/5(theta_ref)
  INTERNAL REFERENCE MODEL ATTITUDE/5(q_ref) -> ERROR CONTROLLER ATTITUDE/2(q_ref)
  ERROR CONTROLLER ATTITUDE/1(pd_ec) -> Sum4/2  "pdd_ec"
  INTERNAL REFERENCE MODEL ATTITUDE/7(phi_ref) -> ERROR CONTROLLER ATTITUDE/4(phi_ref)
  INTERNAL REFERENCE MODEL ATTITUDE/9(psi_ref) -> ERROR CONTROLLER ATTITUDE/6(psi_ref)
  INTERNAL REFERENCE MODEL ATTITUDE/6(r_ref) -> ERROR CONTROLLER ATTITUDE/3(r_ref)
  [T_increment] -> Vector Concatenate/4
  Constant3/1 -> G1+G2/2(G2)
  Constant2/1 -> G1+G2/1(G1)
  Constant9/1 -> G2_comp/1(G2)
  [dv_inner] -> Demux1/1  "dv_inner"
  Sum/1 -> Vector Concatenate2/3
  Demux1/3 -> Scope/1, Sum/1
  Demux1/2 -> Vector Concatenate2/2
  Demux1/1 -> Vector Concatenate2/1
  Demux1/4 -> Vector Concatenate2/4
  Vector Concatenate2/1 -> Matrix Multiply/2
  G2_comp/1(G2_comp) -> Scope/2  "G2_comp"
  Sum5/1 -> Sum17/1
  Saturation1/1 -> ?  "theta_cmd"
  8-shape trajectory/3(psi_traj) -> [psi_traj]
  [Theta_cmd] -> Saturation1/1
  Saturation/1 -> ?  "phi_cmd"
  Sum17/1 -> Sum3/1
  Sum18/1 -> Sum7/1
  Sum19/1 -> Sum9/1
  Constant1/1 -> MATLAB Function1/5(m)
  Demux5/2 -> Sum20/1
  Demux5/1 -> Sum16/1
  [psi_f] -> MATLAB Function1/4(Psi)
  [psi_traj] -> ?
  INTERNAL REFERENCE MODEL VELOCITY/7(X_ref) -> ERROR CONTROLLER VELOCITY/4(X_ref)  "X_ref"
  INTERNAL REFERENCE MODEL VELOCITY/8(Y_ref) -> ERROR CONTROLLER VELOCITY/5(Y_ref)  "Y_ref"
  INTERNAL REFERENCE MODEL VELOCITY/9(Z_ref) -> ERROR CONTROLLER VELOCITY/6(Z_ref)  "Z_ref"
  Doublet Block/1(theta_cmd) -> INTERNAL REFERENCE MODEL ATTITUDE/2(theta_cmd)
  INTERNAL REFERENCE MODEL ATTITUDE/3(rd_ref) -> Sum13/1
  INTERNAL REFERENCE MODEL ATTITUDE/2(qd_ref) -> Sum11/1
  INTERNAL REFERENCE MODEL ATTITUDE/1(pd_ref) -> Sum4/1
  Sum11/1 -> Sum2/1  "qd_des"
  Sum4/1 -> Sum10/1  "pd_des"
  Sum10/1 -> Vector Concatenate/1  "vp"
  Sum2/1 -> Vector Concatenate/2  "vq"
  Sum1/1 -> Vector Concatenate/3  "vr"
  Sum13/1 -> Sum1/1  "rd_des"
  [pd_f] -> Sum10/2
  [qd_f] -> Sum2/2
  [rd_f] -> Sum1/2

== system B5_simulation_paparazzi/Model Block Normal Filters/Continuous Actuator Dynamics ==
  Motor_1_omega_input : Inport
  Motor_2_omega_input : Inport  Port=2
  Motor_3_omega_input : Inport  Port=3
  Motor_4_omega_input : Inport  Port=4
  Butterworth Lowpass 2nd Order1 : Subsystem
  Demux : Demux
  Discrete Transfer Fcn{1..4} (4 alike) : DiscreteTransferFcn  Numerator=[coef_sim_2]  Denominator=[1 coef_sim_1]  SampleTime=sampling_time
  Mux : Mux
  Noise RPM : Subsystem
  Sum : Sum  Inputs=|++
  Transfer Fcn{,1..3} (4 alike) : TransferFcn  Numerator=[omega_des]  Denominator=[1 omega_des]
  omega_1 : Outport
  omega_2 : Outport  Port=2
  omega_3 : Outport  Port=3
  omega_4 : Outport  Port=4
  tag scope: omega_1_f=global, omega_2_f=global, omega_3_f=global, omega_4_f=global
  wires:
  Transfer Fcn3/1 -> omega_4/1  "omega_4"
  Motor_4_omega_input/1 -> Transfer Fcn3/1, Discrete Transfer Fcn4/1  "omega_4_in"
  Motor_3_omega_input/1 -> Transfer Fcn2/1, Discrete Transfer Fcn3/1  "omega_3_in"
  Transfer Fcn1/1 -> omega_2/1  "omega_2"
  Discrete Transfer Fcn2/1 -> Mux/1
  Motor_2_omega_input/1 -> Transfer Fcn1/1, Discrete Transfer Fcn1/1  "omega_2_in"
  Demux/2 -> [omega_2_f]  "omega_2_est"
  Motor_1_omega_input/1 -> Discrete Transfer Fcn2/1, Transfer Fcn/1  "omega_1_in"
  Transfer Fcn/1 -> omega_1/1  "omega_1"
  Demux/4 -> [omega_4_f]  "omega_4_est"
  Discrete Transfer Fcn4/1 -> Mux/4
  Discrete Transfer Fcn1/1 -> Mux/2
  Discrete Transfer Fcn3/1 -> Mux/3
  Transfer Fcn2/1 -> omega_3/1  "omega_3"
  Demux/1 -> [omega_1_f]  "omega_1_est"
  Demux/3 -> [omega_3_f]  "omega_3_est"
  Sum/1 -> Butterworth Lowpass 2nd Order1/1(In)
  Mux/1 -> Sum/1  "pqr_measured"
  Noise RPM/1(Out) -> Sum/2
  Butterworth Lowpass 2nd Order1/1(Out) -> Demux/1

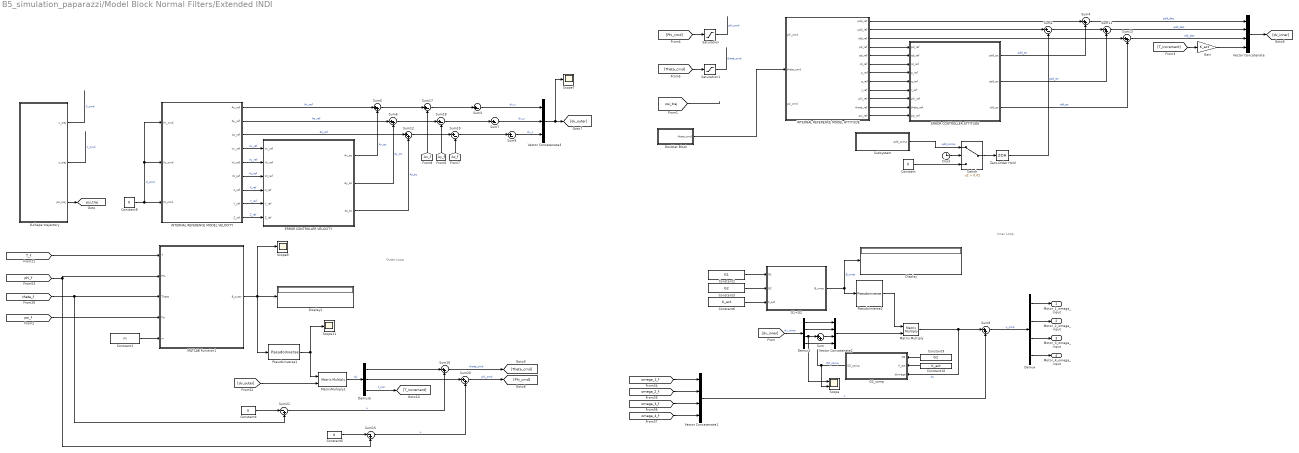
== system B5_simulation_paparazzi/Model Block Normal Filters/Extended INDI ==
  note: Inner Loop
  note: Outer Loop
  8-shape trajectory : Subsystem
  Clock : Clock
  Constant : Constant  Value=0  SampleTime=sampling_time
  Constant1 : Constant  Value=m  SampleTime=sampling_time
  Constant10 : Constant  Value=K_act  SampleTime=sampling_time
  Constant2 : Constant  Value=G1  SampleTime=sampling_time
  Constant3 : Constant  Value=G2  SampleTime=sampling_time
  Constant4 : Constant  Value=0
  Constant5 : Constant  Value=0
  Constant6 : Constant  Value=K_act  SampleTime=sampling_time
  Constant8 : Constant  Value=0  SampleTime=sampling_time
  Constant9 : Constant  Value=G2  SampleTime=sampling_time
  Demux : Demux
  Demux1 : Demux
  Demux5 : Demux  Outputs=3
  Display : Display
  Display1 : Display
  Doublet Block : Subsystem
  ERROR CONTROLLER ATTITUDE : Subsystem
  ERROR CONTROLLER VELOCITY : Subsystem
  G1+G2 : MATLAB Function  TreatAsAtomicUnit=on
  G2_comp : MATLAB Function  TreatAsAtomicUnit=on
  Gain : Gain  Gain=K_act
  INTERNAL REFERENCE MODEL ATTITUDE : Subsystem
  INTERNAL REFERENCE MODEL VELOCITY : Subsystem
  MATLAB Function1 : MATLAB Function  TreatAsAtomicUnit=on
  Matrix Multiply : Product  Multiplication=Matrix(*)
  MatrixMultiply1 : Product  Multiplication=Matrix(*)
  Pseudoinverse1 : dspinverses/Pseudoinverse  wanterr=off  SimulateUsing=Interpreted execution
      settings: SourceProductBaseCode=DS
  Pseudoinverse2 : dspinverses/Pseudoinverse  wanterr=off  SimulateUsing=Interpreted execution
      settings: SourceProductBaseCode=DS
  Saturation : Saturate
  Saturation1 : Saturate
  Scope : Scope  NumInputPorts=2
  Scope11 : Scope
  Scope7 : Scope
  Scope9 : Scope
  Subsystem : Subsystem
  Sum{,4..6,8,11..13,16,20} (10 alike) : Sum  Inputs=|++
  Sum{1,3,7,9,17..19} (7 alike) : Sum  Inputs=|+-
  Sum15 : Sum  Inputs=|-+
  Sum21 : Sum  Inputs=|-+
  Switch : Switch  Criteria=u2 > Threshold  Threshold=0.01
  Vector Concatenate : Concatenate  NumInputs=4
  Vector Concatenate1 : Concatenate  NumInputs=4
  Vector Concatenate2 : Concatenate  NumInputs=4
  Vector Concatenate3 : Concatenate  NumInputs=3
  Zero-Order Hold : ZeroOrderHold  SampleTime=sampling_time
  Motor_1_omega_input : Outport
  Motor_2_omega_input : Outport  Port=2
  Motor_3_omega_input : Outport  Port=3
  Motor_4_omega_input : Outport  Port=4
  tag scope: psi_traj=global
  wires:
  G1+G2/1(B_inner) -> Pseudoinverse2/1, Display/1  "B_inner"
  Vector Concatenate1/1 -> Sum8/2  "u"
  Vector Concatenate/1 -> [dv_inner]
  Matrix Multiply/1 -> G2_comp/3(domega), Sum8/1  "du"
  Demux/1 -> Motor_1_omega_input/1
  [omega_4_f] -> Vector Concatenate1/4
  [omega_2_f] -> Vector Concatenate1/2
  Demux/3 -> Motor_3_omega_input/1
  Sum8/1 -> Demux/1  "u_cmd"
  Pseudoinverse2/1 -> Matrix Multiply/1
  [omega_1_f] -> Vector Concatenate1/1
  Demux/2 -> Motor_2_omega_input/1
  Demux/4 -> Motor_4_omega_input/1
  [omega_3_f] -> Vector Concatenate1/3
  INTERNAL REFERENCE MODEL VELOCITY/5(Vy_ref) -> ERROR CONTROLLER VELOCITY/2(Vy_ref)  "Vy_ref"
  Constant4/1 -> Sum21/1
  Sum16/1 -> [Theta_cmd]  "theta_cmd"
  Sum9/1 -> Vector Concatenate3/3  "dv_z"
  INTERNAL REFERENCE MODEL VELOCITY/2(Ay_ref) -> Sum6/1  "Ay_ref"
  Sum21/1 -> Sum16/2  "u"
  INTERNAL REFERENCE MODEL VELOCITY/6(Vz_ref) -> ERROR CONTROLLER VELOCITY/3(Vz_ref)  "Vz_ref"
  INTERNAL REFERENCE MODEL VELOCITY/4(Vx_ref) -> ERROR CONTROLLER VELOCITY/1(Vx_ref)  "Vx_ref"
  ERROR CONTROLLER VELOCITY/2(Ay_ec) -> Sum6/2  "Ay_ec"
  8-shape trajectory/1(x_traj) -> ?  "X_cmd"
  Sum7/1 -> Vector Concatenate3/2  "dv_y"
  ERROR CONTROLLER VELOCITY/1(Ax_ec) -> Sum5/2  "Ax_ec"
  Sum3/1 -> Vector Concatenate3/1  "dv_x"
  ERROR CONTROLLER VELOCITY/3(Az_ec) -> Sum12/2  "Az_ec"
  Sum12/1 -> Sum19/1
  Constant8/1 -> INTERNAL REFERENCE MODEL VELOCITY/1(Vx_cmd), INTERNAL REFERENCE MODEL VELOCITY/2(Vy_cmd), INTERNAL REFERENCE MODEL VELOCITY/3(Vz_cmd)  "Z_cmd"
  Pseudoinverse1/1 -> Scope11/1, MatrixMultiply1/1
  Sum15/1 -> Sum20/2  "u"
  Vector Concatenate3/1 -> Scope7/1, [dv_outer]
  INTERNAL REFERENCE MODEL VELOCITY/1(Ax_ref) -> Sum5/1  "Ax_ref"
  INTERNAL REFERENCE MODEL VELOCITY/3(Az_ref) -> Sum12/1  "Az_ref"
  Sum20/1 -> [Phi_cmd]  "phi_cmd"
  [T_f] -> MATLAB Function1/1(T)
  Sum6/1 -> Sum18/1
  Constant5/1 -> Sum15/1
  [dv_outer] -> MatrixMultiply1/2
  MATLAB Function1/1(B_outer) -> Scope9/1, Display1/1, Pseudoinverse1/1
  Demux5/3 -> [T_increment]  "t_incr"
  MatrixMultiply1/1 -> Demux5/1  "du"
  8-shape trajectory/2(y_traj) -> ?  "Y_cmd"
  [T_increment] -> Gain/1
  [Ax_f] -> Sum17/2
  [Ay_f] -> Sum18/2
  [Az_f] -> Sum19/2
  [Phi_cmd] -> Saturation/1
  [theta_f] -> Sum21/2, MATLAB Function1/3(Theta)
  [phi_f] -> Sum15/2, MATLAB Function1/2(Phi)
  INTERNAL REFERENCE MODEL ATTITUDE/4(pd_ref) -> ERROR CONTROLLER ATTITUDE/1(pd_ref)
  INTERNAL REFERENCE MODEL ATTITUDE/7(p_ref) -> ERROR CONTROLLER ATTITUDE/4(p_ref)
  ERROR CONTROLLER ATTITUDE/3(rdd_ec) -> Sum13/2  "rdd_ec"
  ERROR CONTROLLER ATTITUDE/2(qdd_ec) -> Sum11/2  "qdd_ec"
  INTERNAL REFERENCE MODEL ATTITUDE/5(qd_ref) -> ERROR CONTROLLER ATTITUDE/2(qd_ref)
  INTERNAL REFERENCE MODEL ATTITUDE/11(theta_ref) -> ERROR CONTROLLER ATTITUDE/8(theta_ref)
  INTERNAL REFERENCE MODEL ATTITUDE/1(pdd_ref) -> Sum4/1
  INTERNAL REFERENCE MODEL ATTITUDE/8(q_ref) -> ERROR CONTROLLER ATTITUDE/5(q_ref)
  ERROR CONTROLLER ATTITUDE/1(pdd_ec) -> Sum4/2  "pdd_ec"
  INTERNAL REFERENCE MODEL ATTITUDE/6(rd_ref) -> ERROR CONTROLLER ATTITUDE/3(rd_ref)
  INTERNAL REFERENCE MODEL ATTITUDE/10(phi_ref) -> ERROR CONTROLLER ATTITUDE/7(phi_ref)
  INTERNAL REFERENCE MODEL ATTITUDE/12(psi_ref) -> ERROR CONTROLLER ATTITUDE/9(psi_ref)
  INTERNAL REFERENCE MODEL ATTITUDE/9(r_ref) -> ERROR CONTROLLER ATTITUDE/6(r_ref)
  Sum13/1 -> Vector Concatenate/3  "rdd_des"
  Sum4/1 -> Vector Concatenate/1  "pdd_des"
  Sum11/1 -> Vector Concatenate/2  "qdd_des"
  Gain/1 -> Vector Concatenate/4
  Constant3/1 -> G1+G2/2(G2)
  Constant6/1 -> G1+G2/3(K_act)
  Constant2/1 -> G1+G2/1(G1)
  Constant9/1 -> G2_comp/1(G2)
  Constant10/1 -> G2_comp/2(K_act)
  [dv_inner] -> Demux1/1  "dv_inner"
  Sum/1 -> Vector Concatenate2/3
  Demux1/3 -> Scope/1, Sum/1
  Demux1/2 -> Vector Concatenate2/2
  Demux1/1 -> Vector Concatenate2/1
  Demux1/4 -> Vector Concatenate2/4
  Vector Concatenate2/1 -> Matrix Multiply/2
  G2_comp/1(G2_comp) -> Scope/2  "G2_comp"
  Sum5/1 -> Sum17/1
  Saturation1/1 -> ?  "theta_cmd"
  INTERNAL REFERENCE MODEL ATTITUDE/2(qdd_ref) -> Sum1/1
  8-shape trajectory/3(psi_traj) -> [psi_traj]
  [Theta_cmd] -> Saturation1/1
  Saturation/1 -> ?  "phi_cmd"
  Sum17/1 -> Sum3/1
  Sum18/1 -> Sum7/1
  Sum19/1 -> Sum9/1
  Constant1/1 -> MATLAB Function1/5(m)
  Demux5/2 -> Sum20/1
  Demux5/1 -> Sum16/1
  [psi_f] -> MATLAB Function1/4(Psi)
  [psi_traj] -> ?
  Clock/1 -> Switch/2
  Constant/1 -> Switch/3
  Switch/1 -> Zero-Order Hold/1
  INTERNAL REFERENCE MODEL VELOCITY/7(X_ref) -> ERROR CONTROLLER VELOCITY/4(X_ref)  "X_ref"
  INTERNAL REFERENCE MODEL VELOCITY/8(Y_ref) -> ERROR CONTROLLER VELOCITY/5(Y_ref)  "Y_ref"
  INTERNAL REFERENCE MODEL VELOCITY/9(Z_ref) -> ERROR CONTROLLER VELOCITY/6(Z_ref)  "Z_ref"
  Doublet Block/1(theta_cmd) -> INTERNAL REFERENCE MODEL ATTITUDE/2(theta_cmd)
  INTERNAL REFERENCE MODEL ATTITUDE/3(rdd_ref) -> Sum13/1
  Subsystem/1(qdd_comp) -> Switch/1  "qdd_comp"
  Sum1/1 -> Sum11/1
  Zero-Order Hold/1 -> Sum1/2

== system B5_simulation_paparazzi/Model Block Normal Filters/Force and Moment Calculation ==
  omega_1 : Inport
  omega_2 : Inport  Port=2
  omega_3 : Inport  Port=3
  omega_4 : Inport  Port=4
  Add : Sum
  Add1 : Sum
  Constant : Constant  Value=0
  Constant1 : Constant  Value=sampling_time  SampleTime=sampling_time
  Constant2 : Constant  Value=G1  SampleTime=sampling_time
  Constant3 : Constant  Value=G2  SampleTime=sampling_time
  Constant5 : Constant  Value=I  SampleTime=sampling_time
  Derivative : Derivative
  Drag Plate Aerodynamics : Subsystem
  Forces due to thrust : MATLAB Function  TreatAsAtomicUnit=on
  Gain : Gain  Gain=0.09
  Gain1 : Gain  Gain=0.09
  Moments due to thrust : MATLAB Function  TreatAsAtomicUnit=on
  Mux : Mux
  Mux1 : Mux  Inputs=3
  Sum : Sum  Inputs=|++
  Moments in body frame : Outport
  Forces in earth frame : Outport  Port=2
  Collective Thrust : Outport  Port=3
  wires:
  Moments due to thrust/1(M_t) -> Add1/2  "thrust_moment_in"
  Constant2/1 -> Forces due to thrust/3(G1), Moments due to thrust/3(G1)
  Constant3/1 -> Moments due to thrust/4(G2)
  omega_4/1 -> Mux/4
  omega_3/1 -> Mux/3
  omega_2/1 -> Mux/2
  omega_1/1 -> Mux/1
  Mux/1 -> Derivative/1, Forces due to thrust/1(omega), Moments due to thrust/1(omega)
  Derivative/1 -> Moments due to thrust/2(omega_dot)
  Constant1/1 -> Moments due to thrust/5(sampling_time)
  [R_bg] -> Forces due to thrust/2(R_bg)
  Forces due to thrust/1(F_t_e) -> Add/2  "thrust_earth"
  Forces due to thrust/2(F_t_b) -> Collective Thrust/1  "thrust_body"
  Add/1 -> Forces in earth frame/1
  Add1/1 -> Moments in body frame/1  "full_moment_in"
  Constant5/1 -> Moments due to thrust/6(I)
  Drag Plate Aerodynamics/1(aero_moment) -> Add1/1  "aero_moment_in"
  Constant/1 -> Mux1/3, Mux1/1
  [theta_cont] -> Gain/1
  [phi_cont] -> Gain1/1
  Gain/1 -> Sum/1
  Gain1/1 -> Sum/2
  Sum/1 -> Mux1/2
  Mux1/1 -> ?  "dummy_moment"
